simulink model "m8_das"  (R2015b)
settings: Solver=FixedStepAuto  SolverMode=SingleTasking  StartTime=0.0  StopTime=10.0  RelTol=1e-3
undefined symbols (not defined in the file): DiscIntNeverNeededParam
libraries: simulink x6
settings Model: Creator=Capstone  LastModifiedBy=muscari.s

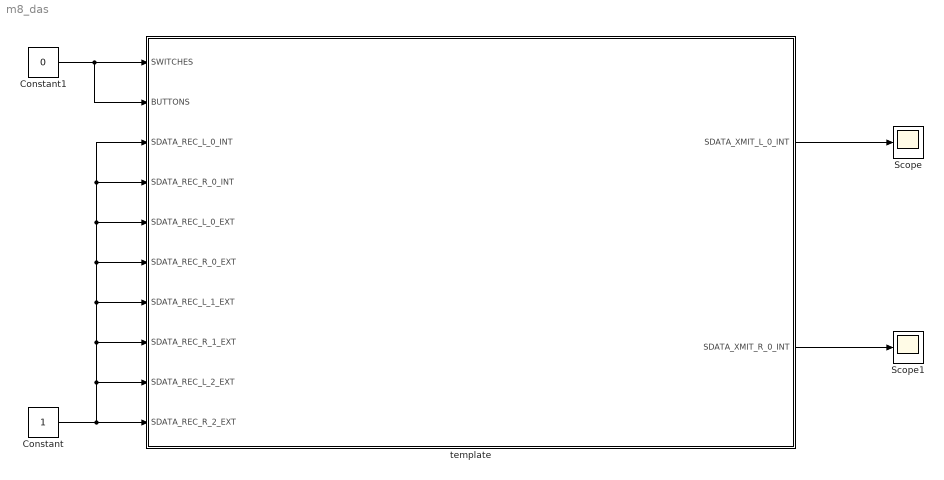
== system m8_das ==
  Constant : Constant  OutDataTypeStr=int32  SampleTime=-1  LockScale=on
  Constant1 : Constant  Value=0  OutDataTypeStr=uint32  SampleTime=-1  LockScale=on
  Scope : Scope
  Scope1 : Scope
  template : Subsystem  TreatAsAtomicUnit=on
  wires:
  template/2(SDATA_XMIT_R_0_INT) -> Scope1/1
  template/1(SDATA_XMIT_L_0_INT) -> Scope/1
  Constant1/1 -> template/1(SWITCHES), template/2(BUTTONS)
  Constant/1 -> template/10(SDATA_REC_R_2_EXT), template/9(SDATA_REC_L_2_EXT), template/8(SDATA_REC_R_1_EXT), template/7(SDATA_REC_L_1_EXT), template/6(SDATA_REC_R_0_EXT), template/5(SDATA_REC_L_0_EXT), template/4(SDATA_REC_R_0_INT), template/3(SDATA_REC_L_0_INT)

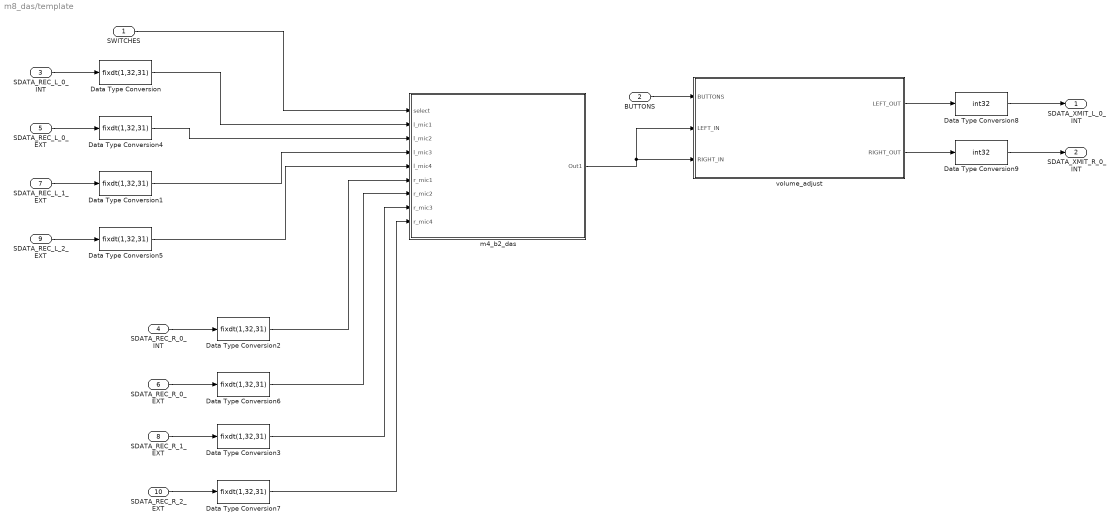
== system m8_das/template ==
  SWITCHES : Inport
  BUTTONS : Inport  Port=2
  SDATA_REC_L_0_INT : Inport  Port=3
  SDATA_REC_R_0_INT : Inport  Port=4
  SDATA_REC_L_0_EXT : Inport  Port=5
  SDATA_REC_R_0_EXT : Inport  Port=6
  SDATA_REC_L_1_EXT : Inport  Port=7
  SDATA_REC_R_1_EXT : Inport  Port=8
  SDATA_REC_L_2_EXT : Inport  Port=9
  SDATA_REC_R_2_EXT : Inport  Port=10
  Data Type Conversion{,1..7} (8 alike) : DataTypeConversion  OutDataTypeStr=fixdt(1,32,31)  ConvertRealWorld=Stored Integer (SI)  RndMeth=Zero
  Data Type Conversion8 : DataTypeConversion  OutDataTypeStr=int32  ConvertRealWorld=Stored Integer (SI)  SaturateOnIntegerOverflow=on  RndMeth=Zero
  Data Type Conversion9 : DataTypeConversion  OutDataTypeStr=int32  ConvertRealWorld=Stored Integer (SI)  SaturateOnIntegerOverflow=on  RndMeth=Zero
  m4_b2_das : Subsystem
  volume_adjust : Subsystem
  SDATA_XMIT_L_0_INT : Outport
  SDATA_XMIT_R_0_INT : Outport  Port=2
  wires:
  SDATA_REC_L_0_INT/1 -> Data Type Conversion/1
  BUTTONS/1 -> volume_adjust/1(BUTTONS)
  volume_adjust/1(LEFT_OUT) -> Data Type Conversion8/1
  volume_adjust/2(RIGHT_OUT) -> Data Type Conversion9/1
  Data Type Conversion8/1 -> SDATA_XMIT_L_0_INT/1
  Data Type Conversion9/1 -> SDATA_XMIT_R_0_INT/1
  Data Type Conversion7/1 -> m4_b2_das/9(r_mic4)
  Data Type Conversion3/1 -> m4_b2_das/8(r_mic3)
  Data Type Conversion6/1 -> m4_b2_das/7(r_mic2)
  Data Type Conversion2/1 -> m4_b2_das/6(r_mic1)
  SWITCHES/1 -> m4_b2_das/1(select)
  Data Type Conversion/1 -> m4_b2_das/2(l_mic1)
  Data Type Conversion4/1 -> m4_b2_das/3(l_mic2)
  Data Type Conversion1/1 -> m4_b2_das/4(l_mic3)
  Data Type Conversion5/1 -> m4_b2_das/5(l_mic4)
  m4_b2_das/1(Out1) -> volume_adjust/2(LEFT_IN), volume_adjust/3(RIGHT_IN)
  SDATA_REC_L_0_EXT/1 -> Data Type Conversion4/1
  SDATA_REC_L_1_EXT/1 -> Data Type Conversion1/1
  SDATA_REC_L_2_EXT/1 -> Data Type Conversion5/1
  SDATA_REC_R_0_INT/1 -> Data Type Conversion2/1
  SDATA_REC_R_0_EXT/1 -> Data Type Conversion6/1
  SDATA_REC_R_1_EXT/1 -> Data Type Conversion3/1
  SDATA_REC_R_2_EXT/1 -> Data Type Conversion7/1

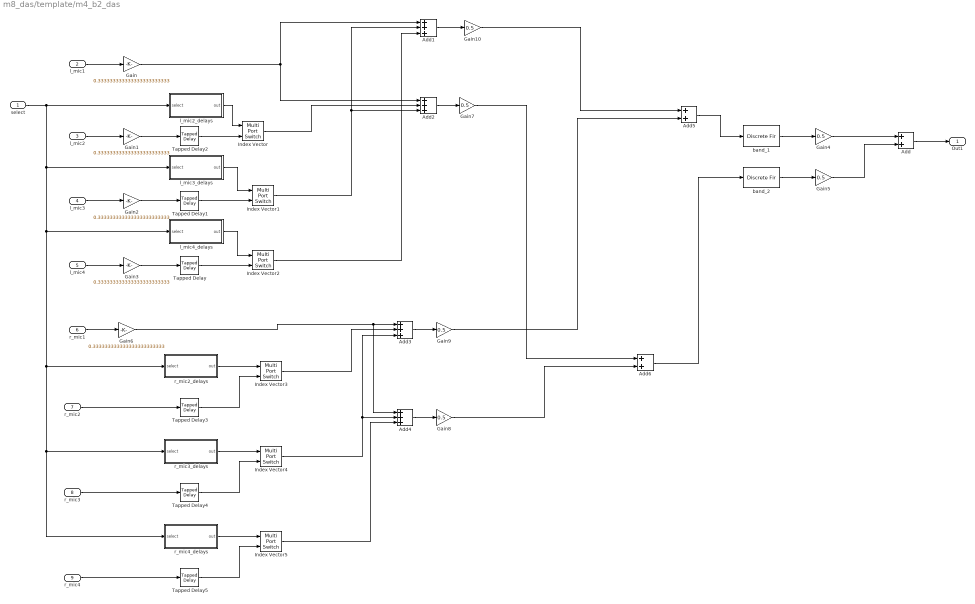
== system m8_das/template/m4_b2_das ==
  select : Inport
  l_mic1 : Inport  Port=2
  l_mic2 : Inport  Port=3
  l_mic3 : Inport  Port=4
  l_mic4 : Inport  Port=5
  r_mic1 : Inport  Port=6
  r_mic2 : Inport  Port=7
  r_mic3 : Inport  Port=8
  r_mic4 : Inport  Port=9
  Add : Sum  OutDataTypeStr=Inherit: Inherit via back propagation  RndMeth=Zero
  Add{1..4} (4 alike) : Sum  Inputs=+++  OutDataTypeStr=Inherit: Inherit via back propagation  RndMeth=Zero
  Add5 : Sum  OutDataTypeStr=Inherit: Inherit via back propagation  RndMeth=Zero
  Add6 : Sum  OutDataTypeStr=Inherit: Inherit via back propagation  RndMeth=Zero
  Gain{,1..3,6} (5 alike) : Gain  Gain=0.333333333333333333333333  ParamDataTypeStr=fixdt(1,32,31)  OutDataTypeStr=Inherit: Inherit via back propagation  RndMeth=Zero
  Gain{4..5,7..10} (6 alike) : Gain  Gain=0.5  ParamDataTypeStr=fixdt(1,32,31)  OutDataTypeStr=Inherit: Inherit via back propagation  RndMeth=Zero
  Index Vector{,1..5} (6 alike) : MultiPortSwitch  DataPortOrder=Zero-based contiguous  Inputs=1  zeroidx=on  OutDataTypeStr=Inherit: Inherit via back propagation  RndMeth=Zero
  Tapped Delay : simulink/Discrete/Tapped Delay  vinit=0.0  samptime=-1  NumDelays=50  DelayOrder=Newest  includeCurrent=on
  Tapped Delay1 : simulink/Discrete/Tapped Delay  vinit=0.0  samptime=-1  NumDelays=25  DelayOrder=Newest  includeCurrent=on
  Tapped Delay2 : simulink/Discrete/Tapped Delay  vinit=0.0  samptime=-1  NumDelays=12  DelayOrder=Newest  includeCurrent=on
  Tapped Delay3 : simulink/Discrete/Tapped Delay  vinit=0.0  samptime=-1  NumDelays=12  DelayOrder=Newest  includeCurrent=on
  Tapped Delay4 : simulink/Discrete/Tapped Delay  vinit=0.0  samptime=-1  NumDelays=25  DelayOrder=Newest  includeCurrent=on
  Tapped Delay5 : simulink/Discrete/Tapped Delay  vinit=0.0  samptime=-1  NumDelays=50  DelayOrder=Newest  includeCurrent=on
  band_1 : DiscreteFir  FilterStructure=Direct form transposed  Coefficients=[-0.00053705791338513377 -0.00044855299737557808 -0.00036099922930643786 -0.00027182738607320795 -0.0001800106196580879 -8.7417645431150305e-05 4.5317422206240127e-19 7.1331751728587471e-05 0.00011027156665220004 9.5221825736704465e-05 0 -0.00020483530962554712 -0.00055007263840206664 -0.0010654350907672839 -0.0017768000544541641 -0.0027032258660805272 -0.0038539915115078267 -0.0052258738517944421 -0.0068008902144789723 -0.0085447214111623055 -0.010406001361532743 -0.012316615678213133 -0.014193095043413446 -0.015939123206432176 -0.017449107952300938 -0.01861269097233053 -0.019320003985495413 -0.019467418420331964 -0.018963488782190799 -0.017734759118407911 -0.01573109041732234 -0.012930175840725469 -0.0093409406089868981 -0.005005573012987645 3.2773545417960019e-18 0.0055672985150007357 0.011558152575777018 0.017809164486738829 0.024137600470880136 0.030348456799490577 0.036242373218319378 0.041624011375338783 0.046310481620462134 0.050139390385166523 0.052976093357513444 0.054719776376280539 0.055308044457367714 0.054719776376280539 0.052976093357513444 0.050139390385166523 0.046310481620462134 0.041624011375338783 0.036242373218319378 0.030348456799490577 0.024137600470880136 0.017809164486738829 0.011558152575777018 0.0055672985150007357 3.2773545417960019e-18 -0.005005573012987645 -0.0093409406089868981 -0.012930175840725469 -0.01573109041732234 -0.017734759118407911 -0.018963488782190799 -0.019467418420331964 -0.019320003985495413 -0.01861269097233053 -0.017449107952300938 -0.015939123206432176 -0.014193095043413446 -0.012316615678213133 -0.010406001361532743 -0.0085447214111623055 -0.0068008902144789723 -0.0052258738517944421 -0.0038539915115078267 -0.0027032258660805272 -0.0017768000544541641 -0.0010654350907672839 -0.00055007263840206664 -0.00020483530962554712 0 9.5221825736704465e-05 0.00011027156665220004 7.1331751728587471e-05 4.5317422206240127e-19 -8.7417645431150305e-05 -0.0001800106196580879 -0.00027182738607320795 -0.00036099922930643786 -0.00044855299737557808 -0.00053705791338513377]  CoefDataTypeStr=fixdt(true,32,31)  ProductDataTypeStr=fixdt(true,32,31)  AccumDataTypeStr=fixdt(true,32,31)  StateDataTypeStr=fixdt(true,32,31)  OutDataTypeStr=fixdt(true,32,31)  RndMeth=Zero
  band_2 : DiscreteFir  FilterStructure=Direct form transposed  Coefficients=[-0.00036313593382457956 -0.00057160558763808358 -0.00065269431705686481 -0.00059959800144019899 -0.00043096011414818828 -0.00020049863435509264 1.1229633857001479e-18 5.2388084292541928e-05 -0.00015767536744401418 -0.00069626860967264841 -0.0015353272375055386 -0.002523852547128952 -0.003394038353231411 -0.0038118140524449097 -0.0034668479487325946 -0.0021807585504879444 2.9770583721313723e-18 0.002762889688022783 0.0055662462194547456 0.0077597235258174448 0.008765948489971127 0.0082756852140677545 0.0063946211523362041 0.0036837282082051439 0.0010588599043410559 -0.00044562265402092087 6.573182092863085e-18 0.002696406106065594 0.007190675726067716 0.012239552123892473 0.016006598436576095 0.016477341145740017 0.012010252700756318 0.0018899011857235338 -0.013271452139196727 -0.031416714103829221 -0.049283952086872938 -0.062989335552494211 -0.068846811086678658 -0.064245745599832149 -0.048375881946775764 -0.022609270700753557 0.0095804797511873496 0.043175729509401982 0.072548299309675754 0.092572998898159897 0.099674944724776851 0.092572998898159897 0.072548299309675754 0.043175729509401982 0.0095804797511873496 -0.022609270700753557 -0.048375881946775764 -0.064245745599832149 -0.068846811086678658 -0.062989335552494211 -0.049283952086872938 -0.031416714103829221 -0.013271452139196727 0.0018899011857235338 0.012010252700756318 0.016477341145740017 0.016006598436576095 0.012239552123892473 0.007190675726067716 0.002696406106065594 6.573182092863085e-18 -0.00044562265402092087 0.0010588599043410559 0.0036837282082051439 0.0063946211523362041 0.0082756852140677545 0.008765948489971127 0.0077597235258174448 0.0055662462194547456 0.002762889688022783 2.9770583721313723e-18 -0.0021807585504879444 -0.0034668479487325946 -0.0038118140524449097 -0.003394038353231411 -0.002523852547128952 -0.0015353272375055386 -0.00069626860967264841 -0.00015767536744401418 5.2388084292541928e-05 1.1229633857001479e-18 -0.00020049863435509264 -0.00043096011414818828 -0.00059959800144019899 -0.00065269431705686481 -0.00057160558763808358 -0.00036313593382457956]  CoefDataTypeStr=fixdt(true,32,31)  ProductDataTypeStr=fixdt(true,32,31)  AccumDataTypeStr=fixdt(true,32,31)  StateDataTypeStr=fixdt(true,32,31)  OutDataTypeStr=fixdt(true,32,31)  RndMeth=Zero
  l_mic2_delays : Subsystem
  l_mic3_delays : Subsystem
  l_mic4_delays : Subsystem
  r_mic2_delays : Subsystem
  r_mic3_delays : Subsystem
  r_mic4_delays : Subsystem
  Out1 : Outport
  wires:
  l_mic1/1 -> Gain/1
  l_mic2/1 -> Gain1/1
  l_mic3/1 -> Gain2/1
  l_mic4/1 -> Gain3/1
  Gain1/1 -> Tapped Delay2/1
  Gain2/1 -> Tapped Delay1/1
  Gain3/1 -> Tapped Delay/1
  Tapped Delay2/1 -> Index Vector/2
  select/1 -> l_mic2_delays/1(select), l_mic3_delays/1(select), r_mic3_delays/1(select), r_mic4_delays/1(select), r_mic2_delays/1(select), l_mic4_delays/1(select)
  Tapped Delay1/1 -> Index Vector1/2
  Tapped Delay/1 -> Index Vector2/2
  Gain/1 -> Add2/1, Add1/1
  Index Vector/1 -> Add2/2
  Index Vector1/1 -> Add1/2, Add2/3
  Index Vector2/1 -> Add1/3
  band_1/1 -> Gain4/1
  band_2/1 -> Gain5/1
  Gain4/1 -> Add/1
  Gain5/1 -> Add/2
  r_mic1/1 -> Gain6/1
  r_mic2/1 -> Tapped Delay3/1
  Tapped Delay3/1 -> Index Vector3/2
  Gain6/1 -> Add3/1, Add4/1
  Index Vector3/1 -> Add3/2
  r_mic3/1 -> Tapped Delay4/1
  Tapped Delay4/1 -> Index Vector4/2
  Index Vector4/1 -> Add3/3, Add4/2
  r_mic4/1 -> Tapped Delay5/1
  Tapped Delay5/1 -> Index Vector5/2
  Index Vector5/1 -> Add4/3
  Add1/1 -> Gain10/1
  Add2/1 -> Gain7/1
  Add/1 -> Out1/1
  Add3/1 -> Gain9/1
  Add4/1 -> Gain8/1
  Add5/1 -> band_1/1
  Add6/1 -> band_2/1
  Gain10/1 -> Add5/1
  Gain9/1 -> Add5/2
  Gain7/1 -> Add6/1
  Gain8/1 -> Add6/2
  l_mic2_delays/1(out) -> Index Vector/1
  l_mic3_delays/1(out) -> Index Vector1/1
  l_mic4_delays/1(out) -> Index Vector2/1
  r_mic2_delays/1(out) -> Index Vector3/1
  r_mic3_delays/1(out) -> Index Vector4/1
  r_mic4_delays/1(out) -> Index Vector5/1

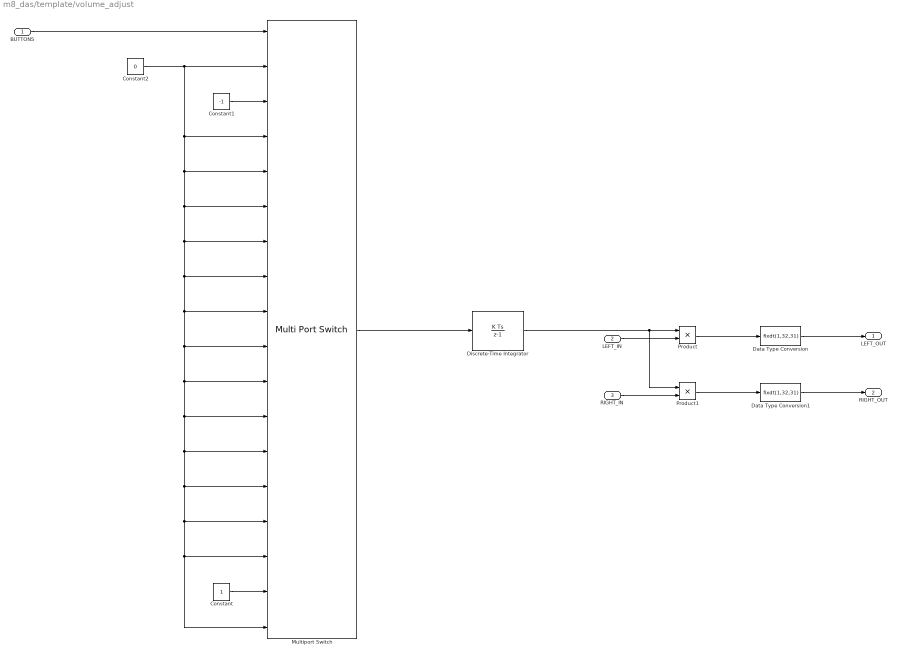
== system m8_das/template/volume_adjust ==
  BUTTONS : Inport
  LEFT_IN : Inport  Port=2
  RIGHT_IN : Inport  Port=3
  Constant : Constant  OutDataTypeStr=fixdt(1,64,31)  SampleTime=-1
  Constant1 : Constant  Value=-1  OutDataTypeStr=fixdt(1,64,31)  SampleTime=-1
  Constant2 : Constant  Value=0  OutDataTypeStr=fixdt(1,64,31)  SampleTime=-1
  Data Type Conversion : DataTypeConversion  OutDataTypeStr=fixdt(1,32,31)  RndMeth=Zero
  Data Type Conversion1 : DataTypeConversion  OutDataTypeStr=fixdt(1,32,31)  RndMeth=Zero
  Discrete-Time Integrator : DiscreteIntegrator  gainval=0.00005  InitialCondition=1  OutDataTypeStr=fixdt(1,64,31)  RndMeth=Zero  SaturateOnIntegerOverflow=on  LimitOutput=on  UpperSaturationLimit=10000  LowerSaturationLimit=0  ICPrevOutput=DiscIntNeverNeededParam  ICPrevScaledInput=DiscIntNeverNeededParam
  Multiport Switch : MultiPortSwitch  Inputs=16  DataPortIndices={16,2}  DataPortForDefault=Additional data port  DiagnosticForDefault=None  OutDataTypeStr=Inherit: Inherit via back propagation  RndMeth=Zero
  Product : Product  OutDataTypeStr=Inherit: Inherit via back propagation  RndMeth=Zero
  Product1 : Product  OutDataTypeStr=Inherit: Inherit via back propagation  RndMeth=Zero
  LEFT_OUT : Outport
  RIGHT_OUT : Outport  Port=2
  wires:
  Multiport Switch/1 -> Discrete-Time Integrator/1
  BUTTONS/1 -> Multiport Switch/1
  Discrete-Time Integrator/1 -> Product1/1, Product/1
  LEFT_IN/1 -> Product/2
  RIGHT_IN/1 -> Product1/2
  Product/1 -> Data Type Conversion/1
  Product1/1 -> Data Type Conversion1/1
  Data Type Conversion/1 -> LEFT_OUT/1
  Data Type Conversion1/1 -> RIGHT_OUT/1
  Constant/1 -> Multiport Switch/17
  Constant1/1 -> Multiport Switch/3
  Constant2/1 -> Multiport Switch/2, Multiport Switch/18, Multiport Switch/16, Multiport Switch/15, Multiport Switch/14, Multiport Switch/13, Multiport Switch/12, Multiport Switch/11, Multiport Switch/10, Multiport Switch/9, Multiport Switch/8, Multiport Switch/7, Multiport Switch/6, Multiport Switch/5, Multiport Switch/4

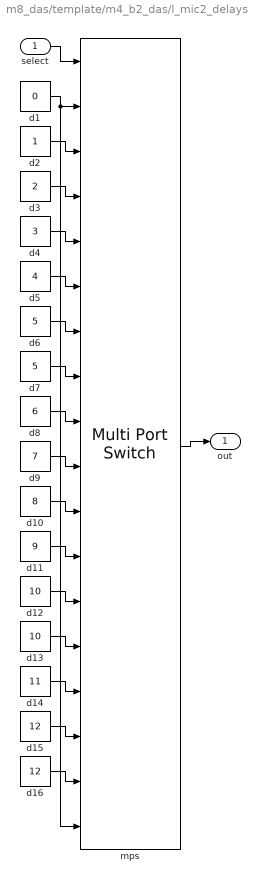
== system m8_das/template/m4_b2_das/l_mic2_delays ==
  select : Inport
  d1 : Constant  Value=0  OutDataTypeStr=uint16  SampleTime=-1
  d10 : Constant  Value=8  OutDataTypeStr=uint16  SampleTime=-1
  d11 : Constant  Value=9  OutDataTypeStr=uint16  SampleTime=-1
  d12 : Constant  Value=10  OutDataTypeStr=uint16  SampleTime=-1
  d13 : Constant  Value=10  OutDataTypeStr=uint16  SampleTime=-1
  d14 : Constant  Value=11  OutDataTypeStr=uint16  SampleTime=-1
  d15 : Constant  Value=12  OutDataTypeStr=uint16  SampleTime=-1
  d16 : Constant  Value=12  OutDataTypeStr=uint16  SampleTime=-1
  d2 : Constant  OutDataTypeStr=uint16  SampleTime=-1
  d3 : Constant  Value=2  OutDataTypeStr=uint16  SampleTime=-1
  d4 : Constant  Value=3  OutDataTypeStr=uint16  SampleTime=-1
  d5 : Constant  Value=4  OutDataTypeStr=uint16  SampleTime=-1
  d6 : Constant  Value=5  OutDataTypeStr=uint16  SampleTime=-1
  d7 : Constant  Value=5  OutDataTypeStr=uint16  SampleTime=-1
  d8 : Constant  Value=6  OutDataTypeStr=uint16  SampleTime=-1
  d9 : Constant  Value=7  OutDataTypeStr=uint16  SampleTime=-1
  mps : MultiPortSwitch  DataPortOrder=Zero-based contiguous  Inputs=16  DataPortForDefault=Additional data port  DiagnosticForDefault=None  OutDataTypeStr=Inherit: Inherit via back propagation  RndMeth=Zero  InputSameDT=on
  out : Outport
  wires:
  select/1 -> mps/1
  mps/1 -> out/1
  d1/1 -> mps/2, mps/18
  d2/1 -> mps/3
  d3/1 -> mps/4
  d4/1 -> mps/5
  d5/1 -> mps/6
  d6/1 -> mps/7
  d7/1 -> mps/8
  d8/1 -> mps/9
  d9/1 -> mps/10
  d10/1 -> mps/11
  d11/1 -> mps/12
  d12/1 -> mps/13
  d13/1 -> mps/14
  d14/1 -> mps/15
  d15/1 -> mps/16
  d16/1 -> mps/17

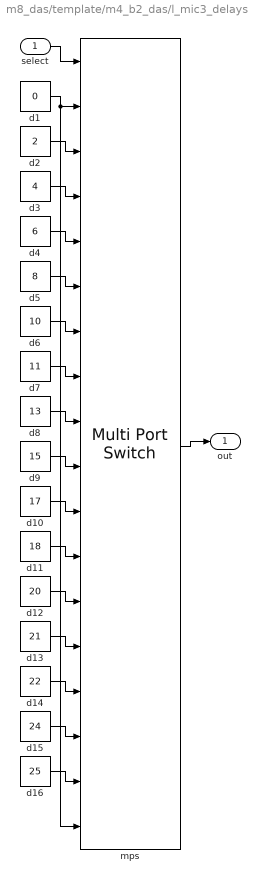
== system m8_das/template/m4_b2_das/l_mic3_delays ==
  select : Inport
  d1 : Constant  Value=0  OutDataTypeStr=uint16  SampleTime=-1
  d10 : Constant  Value=17  OutDataTypeStr=uint16  SampleTime=-1
  d11 : Constant  Value=18  OutDataTypeStr=uint16  SampleTime=-1
  d12 : Constant  Value=20  OutDataTypeStr=uint16  SampleTime=-1
  d13 : Constant  Value=21  OutDataTypeStr=uint16  SampleTime=-1
  d14 : Constant  Value=22  OutDataTypeStr=uint16  SampleTime=-1
  d15 : Constant  Value=24  OutDataTypeStr=uint16  SampleTime=-1
  d16 : Constant  Value=25  OutDataTypeStr=uint16  SampleTime=-1
  d2 : Constant  Value=2  OutDataTypeStr=uint16  SampleTime=-1
  d3 : Constant  Value=4  OutDataTypeStr=uint16  SampleTime=-1
  d4 : Constant  Value=6  OutDataTypeStr=uint16  SampleTime=-1
  d5 : Constant  Value=8  OutDataTypeStr=uint16  SampleTime=-1
  d6 : Constant  Value=10  OutDataTypeStr=uint16  SampleTime=-1
  d7 : Constant  Value=11  OutDataTypeStr=uint16  SampleTime=-1
  d8 : Constant  Value=13  OutDataTypeStr=uint16  SampleTime=-1
  d9 : Constant  Value=15  OutDataTypeStr=uint16  SampleTime=-1
  mps : MultiPortSwitch  DataPortOrder=Zero-based contiguous  Inputs=16  DataPortForDefault=Additional data port  DiagnosticForDefault=None  OutDataTypeStr=Inherit: Inherit via back propagation  RndMeth=Zero  InputSameDT=on
  out : Outport
  wires:
  select/1 -> mps/1
  mps/1 -> out/1
  d1/1 -> mps/2, mps/18
  d2/1 -> mps/3
  d3/1 -> mps/4
  d4/1 -> mps/5
  d5/1 -> mps/6
  d6/1 -> mps/7
  d7/1 -> mps/8
  d8/1 -> mps/9
  d9/1 -> mps/10
  d10/1 -> mps/11
  d11/1 -> mps/12
  d12/1 -> mps/13
  d13/1 -> mps/14
  d14/1 -> mps/15
  d15/1 -> mps/16
  d16/1 -> mps/17

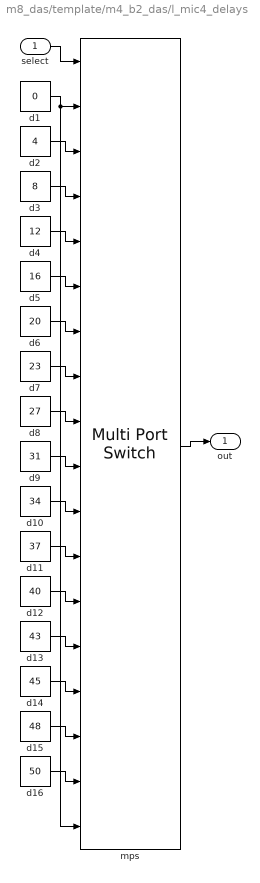
== system m8_das/template/m4_b2_das/l_mic4_delays ==
  select : Inport
  d1 : Constant  Value=0  OutDataTypeStr=uint16  SampleTime=-1
  d10 : Constant  Value=34  OutDataTypeStr=uint16  SampleTime=-1
  d11 : Constant  Value=37  OutDataTypeStr=uint16  SampleTime=-1
  d12 : Constant  Value=40  OutDataTypeStr=uint16  SampleTime=-1
  d13 : Constant  Value=43  OutDataTypeStr=uint16  SampleTime=-1
  d14 : Constant  Value=45  OutDataTypeStr=uint16  SampleTime=-1
  d15 : Constant  Value=48  OutDataTypeStr=uint16  SampleTime=-1
  d16 : Constant  Value=50  OutDataTypeStr=uint16  SampleTime=-1
  d2 : Constant  Value=4  OutDataTypeStr=uint16  SampleTime=-1
  d3 : Constant  Value=8  OutDataTypeStr=uint16  SampleTime=-1
  d4 : Constant  Value=12  OutDataTypeStr=uint16  SampleTime=-1
  d5 : Constant  Value=16  OutDataTypeStr=uint16  SampleTime=-1
  d6 : Constant  Value=20  OutDataTypeStr=uint16  SampleTime=-1
  d7 : Constant  Value=23  OutDataTypeStr=uint16  SampleTime=-1
  d8 : Constant  Value=27  OutDataTypeStr=uint16  SampleTime=-1
  d9 : Constant  Value=31  OutDataTypeStr=uint16  SampleTime=-1
  mps : MultiPortSwitch  DataPortOrder=Zero-based contiguous  Inputs=16  DataPortForDefault=Additional data port  DiagnosticForDefault=None  OutDataTypeStr=Inherit: Inherit via back propagation  RndMeth=Zero  InputSameDT=on
  out : Outport
  wires:
  select/1 -> mps/1
  mps/1 -> out/1
  d1/1 -> mps/2, mps/18
  d2/1 -> mps/3
  d3/1 -> mps/4
  d4/1 -> mps/5
  d5/1 -> mps/6
  d6/1 -> mps/7
  d7/1 -> mps/8
  d8/1 -> mps/9
  d9/1 -> mps/10
  d10/1 -> mps/11
  d11/1 -> mps/12
  d12/1 -> mps/13
  d13/1 -> mps/14
  d14/1 -> mps/15
  d15/1 -> mps/16
  d16/1 -> mps/17

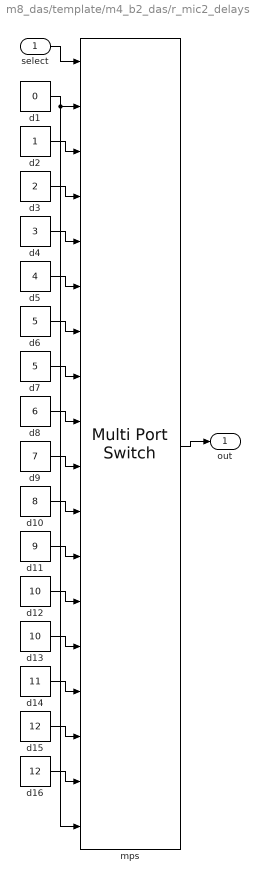
== system m8_das/template/m4_b2_das/r_mic2_delays ==
  select : Inport
  d1 : Constant  Value=0  OutDataTypeStr=uint16  SampleTime=-1
  d10 : Constant  Value=8  OutDataTypeStr=uint16  SampleTime=-1
  d11 : Constant  Value=9  OutDataTypeStr=uint16  SampleTime=-1
  d12 : Constant  Value=10  OutDataTypeStr=uint16  SampleTime=-1
  d13 : Constant  Value=10  OutDataTypeStr=uint16  SampleTime=-1
  d14 : Constant  Value=11  OutDataTypeStr=uint16  SampleTime=-1
  d15 : Constant  Value=12  OutDataTypeStr=uint16  SampleTime=-1
  d16 : Constant  Value=12  OutDataTypeStr=uint16  SampleTime=-1
  d2 : Constant  OutDataTypeStr=uint16  SampleTime=-1
  d3 : Constant  Value=2  OutDataTypeStr=uint16  SampleTime=-1
  d4 : Constant  Value=3  OutDataTypeStr=uint16  SampleTime=-1
  d5 : Constant  Value=4  OutDataTypeStr=uint16  SampleTime=-1
  d6 : Constant  Value=5  OutDataTypeStr=uint16  SampleTime=-1
  d7 : Constant  Value=5  OutDataTypeStr=uint16  SampleTime=-1
  d8 : Constant  Value=6  OutDataTypeStr=uint16  SampleTime=-1
  d9 : Constant  Value=7  OutDataTypeStr=uint16  SampleTime=-1
  mps : MultiPortSwitch  DataPortOrder=Zero-based contiguous  Inputs=16  DataPortForDefault=Additional data port  DiagnosticForDefault=None  OutDataTypeStr=Inherit: Inherit via back propagation  RndMeth=Zero  InputSameDT=on
  out : Outport
  wires:
  select/1 -> mps/1
  mps/1 -> out/1
  d1/1 -> mps/2, mps/18
  d2/1 -> mps/3
  d3/1 -> mps/4
  d4/1 -> mps/5
  d5/1 -> mps/6
  d6/1 -> mps/7
  d7/1 -> mps/8
  d8/1 -> mps/9
  d9/1 -> mps/10
  d10/1 -> mps/11
  d11/1 -> mps/12
  d12/1 -> mps/13
  d13/1 -> mps/14
  d14/1 -> mps/15
  d15/1 -> mps/16
  d16/1 -> mps/17

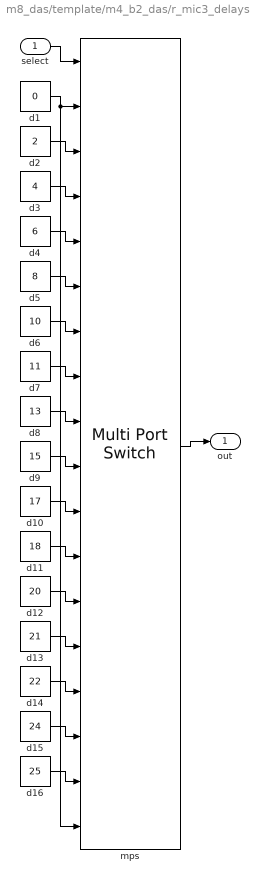
== system m8_das/template/m4_b2_das/r_mic3_delays ==
  select : Inport
  d1 : Constant  Value=0  OutDataTypeStr=uint16  SampleTime=-1
  d10 : Constant  Value=17  OutDataTypeStr=uint16  SampleTime=-1
  d11 : Constant  Value=18  OutDataTypeStr=uint16  SampleTime=-1
  d12 : Constant  Value=20  OutDataTypeStr=uint16  SampleTime=-1
  d13 : Constant  Value=21  OutDataTypeStr=uint16  SampleTime=-1
  d14 : Constant  Value=22  OutDataTypeStr=uint16  SampleTime=-1
  d15 : Constant  Value=24  OutDataTypeStr=uint16  SampleTime=-1
  d16 : Constant  Value=25  OutDataTypeStr=uint16  SampleTime=-1
  d2 : Constant  Value=2  OutDataTypeStr=uint16  SampleTime=-1
  d3 : Constant  Value=4  OutDataTypeStr=uint16  SampleTime=-1
  d4 : Constant  Value=6  OutDataTypeStr=uint16  SampleTime=-1
  d5 : Constant  Value=8  OutDataTypeStr=uint16  SampleTime=-1
  d6 : Constant  Value=10  OutDataTypeStr=uint16  SampleTime=-1
  d7 : Constant  Value=11  OutDataTypeStr=uint16  SampleTime=-1
  d8 : Constant  Value=13  OutDataTypeStr=uint16  SampleTime=-1
  d9 : Constant  Value=15  OutDataTypeStr=uint16  SampleTime=-1
  mps : MultiPortSwitch  DataPortOrder=Zero-based contiguous  Inputs=16  DataPortForDefault=Additional data port  DiagnosticForDefault=None  OutDataTypeStr=Inherit: Inherit via back propagation  RndMeth=Zero  InputSameDT=on
  out : Outport
  wires:
  select/1 -> mps/1
  mps/1 -> out/1
  d1/1 -> mps/2, mps/18
  d2/1 -> mps/3
  d3/1 -> mps/4
  d4/1 -> mps/5
  d5/1 -> mps/6
  d6/1 -> mps/7
  d7/1 -> mps/8
  d8/1 -> mps/9
  d9/1 -> mps/10
  d10/1 -> mps/11
  d11/1 -> mps/12
  d12/1 -> mps/13
  d13/1 -> mps/14
  d14/1 -> mps/15
  d15/1 -> mps/16
  d16/1 -> mps/17

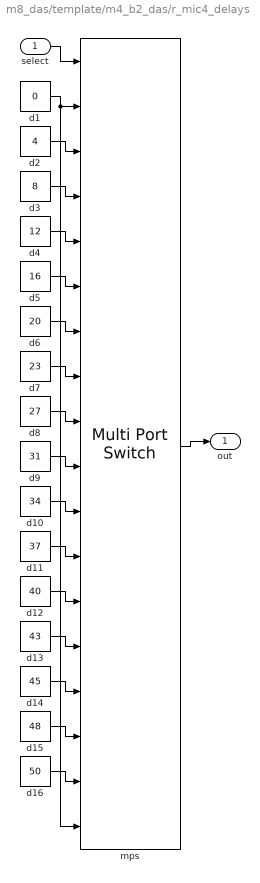
== system m8_das/template/m4_b2_das/r_mic4_delays ==
  select : Inport
  d1 : Constant  Value=0  OutDataTypeStr=uint16  SampleTime=-1
  d10 : Constant  Value=34  OutDataTypeStr=uint16  SampleTime=-1
  d11 : Constant  Value=37  OutDataTypeStr=uint16  SampleTime=-1
  d12 : Constant  Value=40  OutDataTypeStr=uint16  SampleTime=-1
  d13 : Constant  Value=43  OutDataTypeStr=uint16  SampleTime=-1
  d14 : Constant  Value=45  OutDataTypeStr=uint16  SampleTime=-1
  d15 : Constant  Value=48  OutDataTypeStr=uint16  SampleTime=-1
  d16 : Constant  Value=50  OutDataTypeStr=uint16  SampleTime=-1
  d2 : Constant  Value=4  OutDataTypeStr=uint16  SampleTime=-1
  d3 : Constant  Value=8  OutDataTypeStr=uint16  SampleTime=-1
  d4 : Constant  Value=12  OutDataTypeStr=uint16  SampleTime=-1
  d5 : Constant  Value=16  OutDataTypeStr=uint16  SampleTime=-1
  d6 : Constant  Value=20  OutDataTypeStr=uint16  SampleTime=-1
  d7 : Constant  Value=23  OutDataTypeStr=uint16  SampleTime=-1
  d8 : Constant  Value=27  OutDataTypeStr=uint16  SampleTime=-1
  d9 : Constant  Value=31  OutDataTypeStr=uint16  SampleTime=-1
  mps : MultiPortSwitch  DataPortOrder=Zero-based contiguous  Inputs=16  DataPortForDefault=Additional data port  DiagnosticForDefault=None  OutDataTypeStr=Inherit: Inherit via back propagation  RndMeth=Zero  InputSameDT=on
  out : Outport
  wires:
  select/1 -> mps/1
  mps/1 -> out/1
  d1/1 -> mps/2, mps/18
  d2/1 -> mps/3
  d3/1 -> mps/4
  d4/1 -> mps/5
  d5/1 -> mps/6
  d6/1 -> mps/7
  d7/1 -> mps/8
  d8/1 -> mps/9
  d9/1 -> mps/10
  d10/1 -> mps/11
  d11/1 -> mps/12
  d12/1 -> mps/13
  d13/1 -> mps/14
  d14/1 -> mps/15
  d15/1 -> mps/16
  d16/1 -> mps/17
